simulink model "q_srv02_lab2_mdl"  (Simulink 10.2)
settings: Solver=ode1  StartTime=0.0  StopTime=inf  FixedStep=0.001  RelTol=1e-3  AbsTol=1e-6  EnableMultiTasking=on
values from neighbouring files (symbols this model uses):
  K = Am / Beq_v    [d_model_param.m]    (also in setup_srv02_lab2_mdl.m = 1)
  K_AMP = 1    [setup_srv02_lab2_mdl.m]
  tau = Jeq / Beq_v    [d_model_param.m]    (also in setup_srv02_lab2_mdl.m = 0.1)
  VMAX_DAC = 10    [setup_srv02_lab2_mdl.m]
  wcf_e = 2 * pi * 25.0    (= 157.079632679)    [setup_srv02_lab2_mdl.m]
  zetaf_e = 0.9    [setup_srv02_lab2_mdl.m]
undefined symbols (not defined in the file or in its folder): HIL, K_ENC, K_POT, K_TACH, qc_get_step_size, VMAX_AMP
libraries: quarc_library x6, simulink x2
settings Model: Creator=MLevis  LastModifiedBy=temami  SimulationMode=external  ExtModeTrigDuration=10000
settings SolverCC: AutoScaleAbsTol=off  PositivePriorityOrder=on
settings OptimizationCC: BlockReduction=off  BooleanDataType=off  OptimizeBlockIOStorage=off  BufferReuse=off  GlobalBufferReuse=off  ExpressionFolding=off  ExpressionDepthLimit=2147483647  LocalBlockOutputs=off  InitFltsAndDblsToZero=on  OptimizeDataStoreBuffers=off  BusAssignmentInplaceUpdate=off
settings DebuggingCC: SaveWithParameterizedLinksMsg=none  SignalResolutionControl=TryResolveAllWithWarning  MultiTaskDSMMsg=warning  MultiTaskCondExecSysMsg=none  StateNameClashWarn=warning
settings HardwareCC: TargetHWDeviceType=32-bit Generic
settings RTWCC: Description=QUARC Win64 Target  SystemTargetFile=quarc_win64.tlc  TemplateMakefile=quarc_default_tmf
settings STFCustomTargetCC: TargetPreCompLibLocation=C:\PROGRA~3\QUARC\lib\2020b\win64\release  ConcurrentExecutionCompliant=on  CPPClassGenCompliant=on  SystemTargetFile=quarc_win64.tlc
settings GRTTargetCC: TargetPreCompLibLocation=C:\PROGRA~3\QUARC\lib\2020b\win64\release  ParMdlRefBuildCompliant=off  CompOptLevelCompliant=off  MatFileLogging=off  UseToolchainInfoCompliant=off  ExtMode=on  ExtModeMexFile=quarc_comm

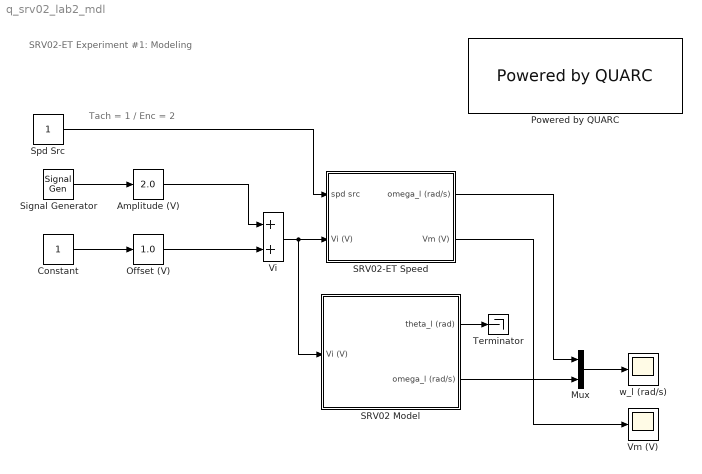
== system q_srv02_lab2_mdl ==
  note: SRV02-ET Experiment #1: Modeling
  note: Tach = 1 / Enc = 2
  Amplitude (V) : simulink/Math Operations/Slider Gain  gain=2.0  low=0  high=5
  Constant : Constant
  Mux : Mux  Inputs=2
  Offset (V) : simulink/Math Operations/Slider Gain  gain=1.0  low=-5  high=5
  Powered by QUARC : quarc_library/Logos/Powered by QUARC
  SRV02 Model : Subsystem
  SRV02-ET Speed : Subsystem
  Signal Generator : SignalGenerator  WaveForm=square
  Spd Src : Constant
  Terminator : Terminator
  Vi : Sum
  Vm (V) : Scope
  w_l (rad/s) : Scope
  wires:
  Constant/1 -> Offset (V)/1
  Offset (V)/1 -> Vi/2
  Vi/1 -> SRV02 Model/1(Vi (V)), SRV02-ET Speed/2(Vi (V))
  Mux/1 -> w_l (rad/s)/1
  SRV02-ET Speed/2(Vm (V)) -> Vm (V)/1
  SRV02 Model/2(omega_l (rad/s)) -> Mux/2
  SRV02-ET Speed/1(omega_l (rad/s)) -> Mux/1
  SRV02 Model/1(theta_l (rad)) -> Terminator/1
  Signal Generator/1 -> Amplitude (V)/1
  Amplitude (V)/1 -> Vi/1
  Spd Src/1 -> SRV02-ET Speed/1(spd src)

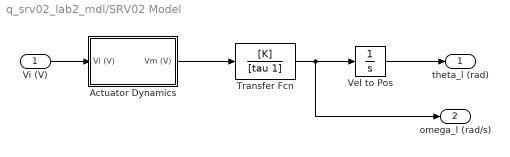
== system q_srv02_lab2_mdl/SRV02 Model ==
  Vi (V) : Inport
  Actuator Dynamics : Subsystem
  Transfer Fcn : TransferFcn  Numerator=[K]  Denominator=[tau 1]
  Vel to Pos : Integrator
  theta_l (rad) : Outport  VectorParamsAs1DForOutWhenUnconnected=off
  omega_l (rad/s) : Outport  Port=2  VectorParamsAs1DForOutWhenUnconnected=off
  wires:
  Vi (V)/1 -> Actuator Dynamics/1(Vi (V))
  Actuator Dynamics/1(Vm (V)) -> Transfer Fcn/1
  Vel to Pos/1 -> theta_l (rad)/1
  Transfer Fcn/1 -> Vel to Pos/1, omega_l (rad/s)/1

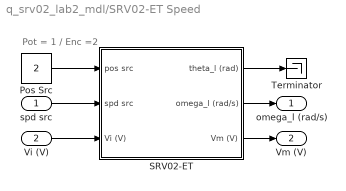
== system q_srv02_lab2_mdl/SRV02-ET Speed ==
  note: Pot = 1 / Enc =2
  spd src : Inport
  Vi (V) : Inport  Port=2
  Pos Src : Constant  Value=2
  SRV02-ET : Subsystem
  Terminator : Terminator
  omega_l (rad/s) : Outport  VectorParamsAs1DForOutWhenUnconnected=off
  Vm (V) : Outport  Port=2  VectorParamsAs1DForOutWhenUnconnected=off
  wires:
  SRV02-ET/3(Vm (V)) -> Vm (V)/1
  Vi (V)/1 -> SRV02-ET/3(Vi (V))
  SRV02-ET/2(omega_l (rad/s)) -> omega_l (rad/s)/1
  spd src/1 -> SRV02-ET/2(spd src)
  SRV02-ET/1(theta_l (rad)) -> Terminator/1
  Pos Src/1 -> SRV02-ET/1(pos src)

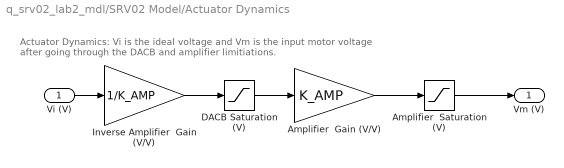
== system q_srv02_lab2_mdl/SRV02 Model/Actuator Dynamics ==
  note: Actuator Dynamics: Vi is the ideal voltage and Vm is the
      | input motor voltage after going through the DACB and amplifier limitiations.
  Vi (V) : Inport
  Amplifier  Gain (V/V) : Gain  Gain=K_AMP
  Amplifier  Saturation (V) : Saturate  UpperLimit=VMAX_AMP  LowerLimit=-VMAX_AMP
  DACB Saturation (V) : Saturate  UpperLimit=VMAX_DAC  LowerLimit=-VMAX_DAC
  Inverse Amplifier  Gain (V/V) : Gain  Gain=1/K_AMP
  Vm (V) : Outport  VectorParamsAs1DForOutWhenUnconnected=off
  wires:
  Inverse Amplifier  Gain (V/V)/1 -> DACB Saturation (V)/1
  DACB Saturation (V)/1 -> Amplifier  Gain (V/V)/1
  Amplifier  Gain (V/V)/1 -> Amplifier  Saturation (V)/1
  Vi (V)/1 -> Inverse Amplifier  Gain (V/V)/1
  Amplifier  Saturation (V)/1 -> Vm (V)/1

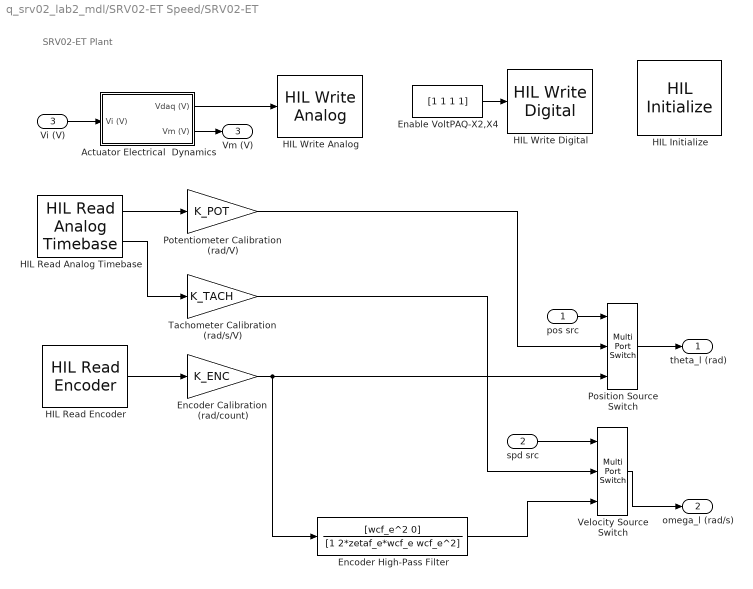
== system q_srv02_lab2_mdl/SRV02-ET Speed/SRV02-ET ==
  note: SRV02-ET Plant
  pos src : Inport
  spd src : Inport  Port=2
  Vi (V) : Inport  Port=3
  Actuator Electrical  Dynamics : Subsystem
  Enable VoltPAQ-X2,X4 : Constant  Value=[1 1 1 1]
  Encoder Calibration  (rad/count) : Gain  Gain=K_ENC  SaturateOnIntegerOverflow=on  OutDataTypeStr=Inherit: Same as input  ParamDataTypeStr=Inherit: Same as input
  Encoder High-Pass Filter : TransferFcn  Numerator=[wcf_e^2 0]  Denominator=[1 2*zetaf_e*wcf_e wcf_e^2]
  HIL Initialize : quarc_library/Data Acquisition/Generic/Configuration/HIL Initialize  object_name=HIL-1  board_type=q2_usb  board_number=0  board_options=d0=digital;d1=digital;led=auto;update_rate=normal;decimation=1  exclusive=off  active=off  hardware_clocks=[0]  clock_modes=[]  initial_clock_frequencies=[]  set_clock_params_at_start=off  set_clock_params_at_switch_in=off  set_clock_frequencies_at_start=off  set_clock_frequencies_at_switch_in=off  analog_input_channels=[0:1]  analog_input_configurations=[]  analog_input_maximums=10  analog_input_minimums=-10  set_analog_input_params_at_start=on  set_analog_input_params_at_switch_in=off  analog_output_channels=[0:1]  analog_output_maximums=10  analog_output_minimums=-10  initial_analog_outputs=[0]  final_analog_outputs=[0]  watchdog_analog_outputs=0  set_analog_output_params_at_start=on  set_analog_output_params_at_switch_in=off  set_analog_outputs_at_start=on  set_analog_outputs_at_switch_in=off  set_analog_outputs_at_terminate=on  set_analog_outputs_at_switch_out=off  set_analog_outputs_on_watchdog=off  digital_input_channels=[]  digital_output_channels=[]  digital_output_configuration=[]  initial_digital_outputs=[1]  final_digital_outputs=[1]  watchdog_digital_outputs=[1]  set_digital_output_params_at_start=off  set_digital_output_params_at_switch_in=off  set_digital_outputs_at_start=on  set_digital_outputs_at_switch_in=off  set_digital_outputs_at_terminate=on  set_digital_outputs_at_switch_out=off  set_digital_outputs_on_watchdog=off  encoder_channels=[0:1]  quadrature=[4]  encoder_filter_frequency=[]  initial_encoder_counts=[0]  set_encoder_params_at_start=on  set_encoder_params_at_switch_in=off  set_encoder_counts_at_start=on  set_encoder_counts_at_switch_in=off  pwm_channels=[]  pwm_modes=[0]  pwm_frequency=1/0.020  pwm_configuration=[]  pwm_alignment=[]  pwm_polarity=[]  pwm_leading_deadband=[]  pwm_trailing_deadband=[]  initial_pwm_outputs=[0]  final_pwm_outputs=[0]  watchdog_pwm_outputs=[0]  set_pwm_params_at_start=on  set_pwm_params_at_switch_in=off  set_pwm_outputs_at_start=on  set_pwm_outputs_at_switch_in=off  set_pwm_outputs_at_terminate=on  set_pwm_outputs_at_switch_out=off  set_pwm_outputs_on_watchdog=off  other_output_channels=[]  initial_other_outputs=[]  final_other_outputs=[]  watchdog_other_outputs=[]  set_other_outputs_at_start=off  set_other_outputs_at_switch_in=off  set_other_outputs_at_terminate=off  set_other_outputs_at_switch_out=off  set_other_outputs_on_watchdog=off
  HIL Read Analog Timebase : quarc_library/Data Acquisition/Generic/Timebases/HIL Read Analog Timebase  Tag=unassigned  object_name=HIL-1  channels=[0:1]  clock=0  active=on  vector_output=off  overflow_mode=Error on overflow  samples_in_buffer=max(ceil(1/qc_get_step_size), 1)
      settings: AttributesFormatString=(%<object_name>)  SourceProductName=QUARC Targets
  HIL Read Encoder : quarc_library/Data Acquisition/Generic/Immediate I//O/HIL Read Encoder  Tag=unassigned  object_name=HIL-1  channels=0  sample_time=qc_get_step_size  active=on  vector_output=off  data_type_mode=Inherit via back propagation  data_type=double
  HIL Write Analog : quarc_library/Data Acquisition/Generic/Immediate I//O/HIL Write Analog  Tag=unassigned  object_name=HIL-1  channels=0  sample_time=-1  active=off  vector_input=off
  HIL Write Digital : quarc_library/Data Acquisition/Generic/Immediate I//O/HIL Write Digital  object_name=HIL-1  channels=[0:3]  sample_time=-1  active=off  vector_input=on
      settings: SourceProductName=QUARC Targets
  Position Source Switch : MultiPortSwitch  Inputs=2
  Potentiometer Calibration  (rad/V) : Gain  Gain=K_POT  SaturateOnIntegerOverflow=on  OutDataTypeStr=Inherit: Same as input  ParamDataTypeStr=Inherit: Same as input
  Tachometer Calibration  (rad/s/V) : Gain  Gain=K_TACH  SaturateOnIntegerOverflow=on  OutDataTypeStr=Inherit: Same as input  ParamDataTypeStr=Inherit: Same as input
  Velocity Source Switch : MultiPortSwitch  Inputs=2
  theta_l (rad) : Outport  InitialOutput=0  VectorParamsAs1DForOutWhenUnconnected=off
  omega_l (rad/s) : Outport  Port=2  InitialOutput=0  VectorParamsAs1DForOutWhenUnconnected=off
  Vm (V) : Outport  Port=3  InitialOutput=0  VectorParamsAs1DForOutWhenUnconnected=off
  wires:
  HIL Read Analog Timebase/2 -> Tachometer Calibration  (rad/s/V)/1
  HIL Read Encoder/1 -> Encoder Calibration  (rad/count)/1
  Potentiometer Calibration  (rad/V)/1 -> Position Source Switch/2
  spd src/1 -> Velocity Source Switch/1
  pos src/1 -> Position Source Switch/1
  Position Source Switch/1 -> theta_l (rad)/1
  Velocity Source Switch/1 -> omega_l (rad/s)/1
  Actuator Electrical  Dynamics/2(Vm (V)) -> Vm (V)/1
  Actuator Electrical  Dynamics/1(Vdaq (V)) -> HIL Write Analog/1
  HIL Read Analog Timebase/1 -> Potentiometer Calibration  (rad/V)/1
  Vi (V)/1 -> Actuator Electrical  Dynamics/1(Vi (V))
  Encoder Calibration  (rad/count)/1 -> Encoder High-Pass Filter/1, Position Source Switch/3
  Tachometer Calibration  (rad/s/V)/1 -> Velocity Source Switch/2
  Enable VoltPAQ-X2,X4/1 -> HIL Write Digital/1
  Encoder High-Pass Filter/1 -> Velocity Source Switch/3

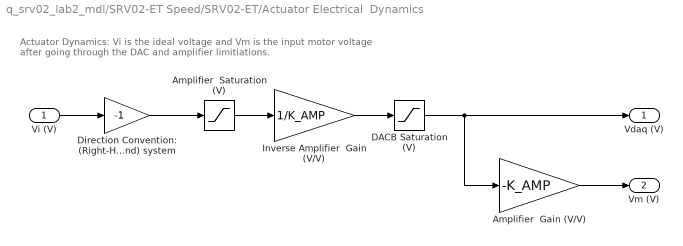
== system q_srv02_lab2_mdl/SRV02-ET Speed/SRV02-ET/Actuator Electrical  Dynamics ==
  note: Actuator Dynamics: Vi is the ideal voltage and Vm is the
      | input motor voltage after going through the DAC and amplifier limitiations.
  Vi (V) : Inport
  Amplifier  Gain (V/V) : Gain  Gain=-K_AMP
  Amplifier  Saturation (V) : Saturate  UpperLimit=VMAX_AMP  LowerLimit=-VMAX_AMP
  DACB Saturation (V) : Saturate  UpperLimit=VMAX_DAC  LowerLimit=-VMAX_DAC
  Direction Convention: (Right-Hand) system : Gain  Gain=-1  SaturateOnIntegerOverflow=on  OutDataTypeStr=Inherit: Same as input  ParamDataTypeStr=Inherit: Same as input
  Inverse Amplifier  Gain (V/V) : Gain  Gain=1/K_AMP
  Vdaq (V) : Outport  VectorParamsAs1DForOutWhenUnconnected=off
  Vm (V) : Outport  Port=2  VectorParamsAs1DForOutWhenUnconnected=off
  wires:
  Vi (V)/1 -> Direction Convention: (Right-Hand) system/1
  Amplifier  Saturation (V)/1 -> Inverse Amplifier  Gain (V/V)/1
  Inverse Amplifier  Gain (V/V)/1 -> DACB Saturation (V)/1
  DACB Saturation (V)/1 -> Amplifier  Gain (V/V)/1, Vdaq (V)/1
  Amplifier  Gain (V/V)/1 -> Vm (V)/1
  Direction Convention: (Right-Hand) system/1 -> Amplifier  Saturation (V)/1
